simulink model "lr5"  (R2023b)
settings: Solver=FixedStepAuto  StartTime=0.0  StopTime=100  FixedStep=1e-2  RelTol=1e-3
libraries: instrumentseriallib x2
settings Model: Creator=User  LastModifiedBy=deniskirbaba
settings ModelReferenceCC: EnableRefExpFcnMdlSchedulingChecks=on

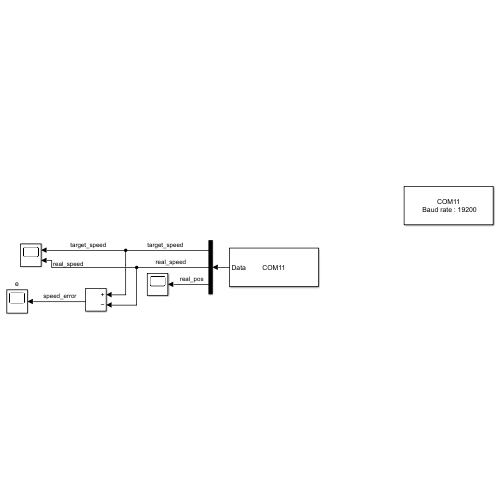
[thumbnail: Simulink's stored preview of the top-level diagram]
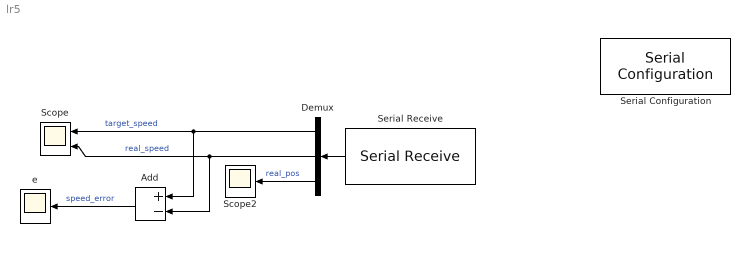
== system lr5 ==
  Add : Sum  Inputs=+-
  Demux : Demux  Outputs=3
  Scope : Scope  NumInputPorts=2
  Scope2 : Scope
  Serial Configuration : instrumentseriallib/Serial Configuration  Priority=-200000  PortSel=COM11  Port=COM11  ComPort=COM11  BaudRate=19200  DataBits=8  Parity=none  StopBits=1  ByteOrder=little-endian  FlowControl=none  Timeout=10  SimulateUsing=Interpreted execution  BlockInModel=on  aMode=1
  Serial Receive : instrumentseriallib/Serial Receive  Priority=1  PortSel=COM11  Port=COM11  ComPort=COM11  DataType=single  SaveDataType=uint8  ToggleHeader=on  Header='N'  ToggleTerminator=on  Terminator=Custom terminator  CustomTerminator='E'  InputFormat=Column major  ToggleDataSize=on  DataSize=3  EnableBlockingMode=on  ActionDataUnavailable=Output custom value  ActionWhenDataUnavailable=Output custom value  CustomValue=-1  SampleTime=0.01  SimulateUsing=Interpreted execution  BlockInModel=on  aMode=1
  e : Scope
  wires:
  Serial Receive/1 -> Demux/1
  Demux/1 -> Add/1, Scope/1  "target_speed"
  Demux/2 -> Add/2, Scope/2  "real_speed"
  Demux/3 -> Scope2/1  "real_pos"
  Add/1 -> e/1  "speed_error"
